simulink model "week1"  (R2020b)
settings: Solver=VariableStepAuto  StartTime=0.0  StopTime=10.0  RelTol=1e-3
settings Model: Creator=hp  LastModifiedBy=hp

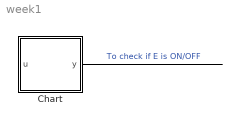
== system week1 ==
  Chart : Stateflow chart  TreatAsAtomicUnit=on
  wires:
  ? -> Chart/1(u)  "E_ON/OFF"
  Chart/1(y) -> ?  "To check if E is ON/OFF"

== stateflow chart week1/Chart ==
  state Elevator_on
    entry: y=1;
  state Elevator_off
    entry: y=0;
  (default) -> Elevator_on
  Elevator_on -> Elevator_off : [u==0]
  Elevator_off -> Elevator_on : [u==1]
  data: u input; y output
